simulink model "JK_flipflop_masterslave"  (R2020a)
settings: Solver=VariableStepAuto  StartTime=0.0  StopTime=inf  RelTol=1e-3
libraries: simulink_extras x1
settings Model: EnablePacing=on  Creator=F1  LastModifiedBy=F1

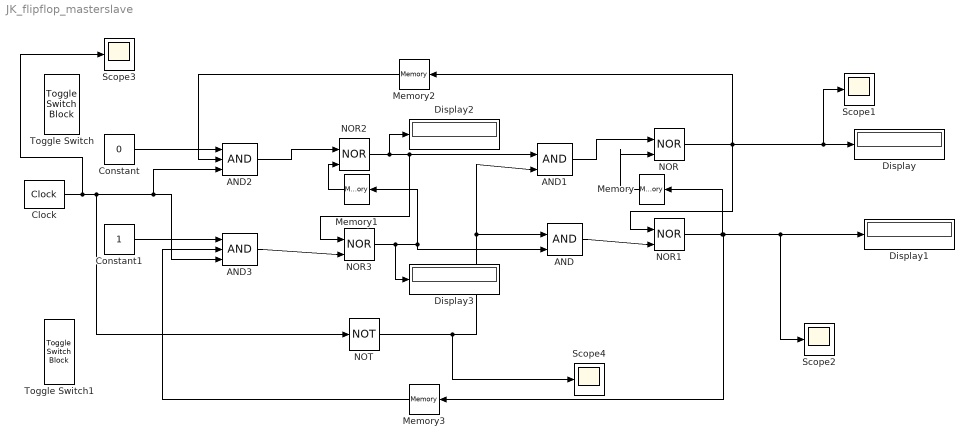
== system JK_flipflop_masterslave ==
  AND : Logic  IconShape=distinctive  AllPortsSameDT=off  OutDataTypeStr=boolean
  AND1 : Logic  IconShape=distinctive  AllPortsSameDT=off  OutDataTypeStr=boolean
  AND2 : Logic  Inputs=3  IconShape=distinctive  AllPortsSameDT=off  OutDataTypeStr=boolean
  AND3 : Logic  Inputs=3  IconShape=distinctive  AllPortsSameDT=off  OutDataTypeStr=boolean
  Clock : simulink_extras/Flip Flops/Clock  period=2
  Constant : Constant  Value=0
  Constant1 : Constant
  Display{,1..3} (4 alike) : Display
  Memory{,1..3} (4 alike) : Memory
  NOR{,1..3} (4 alike) : Logic  Operator=NOR  IconShape=distinctive  AllPortsSameDT=off  OutDataTypeStr=boolean
  NOT : Logic  Operator=NOT  IconShape=distinctive  AllPortsSameDT=off  OutDataTypeStr=boolean
  Scope{1..4} (4 alike) : Scope
  Toggle Switch : ToggleSwitchBlock
      settings: Values={{'Off', 'On'}, [0 1]}
  Toggle Switch1 : ToggleSwitchBlock
      settings: Values={{'Off', 'On'}, [0 1]}
  wires:
  NOR2/1 -> NOR3/1, AND1/1, Display2/1
  AND3/1 -> NOR3/2
  NOR3/1 -> Display3/1, AND/2, Memory1/1
  Constant/1 -> AND2/1
  Constant1/1 -> AND3/1
  Clock/1 -> Scope3/1, AND3/3, AND2/3, NOT/1
  Memory/1 -> NOR/2
  Memory1/1 -> NOR2/2
  NOR/1 -> Memory2/1, Scope1/1, Display/1, NOR1/1
  NOR1/1 -> Memory/1, Memory3/1, Display1/1, Scope2/1
  NOT/1 -> Scope4/1, AND1/2, AND/1
  AND/1 -> NOR1/2
  AND1/1 -> NOR/1
  AND2/1 -> NOR2/1
  Memory2/1 -> AND2/2
  Memory3/1 -> AND3/2
